simulink model "sampleModel1496_4"  (R2023a)
settings: Solver=VariableStepAuto  StartTime=0.0  StopTime=10.0  RelTol=1e-3
libraries: hdlsllib x6
settings Model: Creator=user1  LastModifiedBy=user1

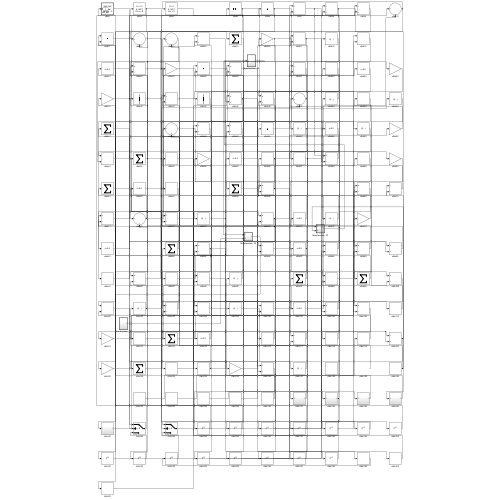
[thumbnail: Simulink's stored preview of the top-level diagram]
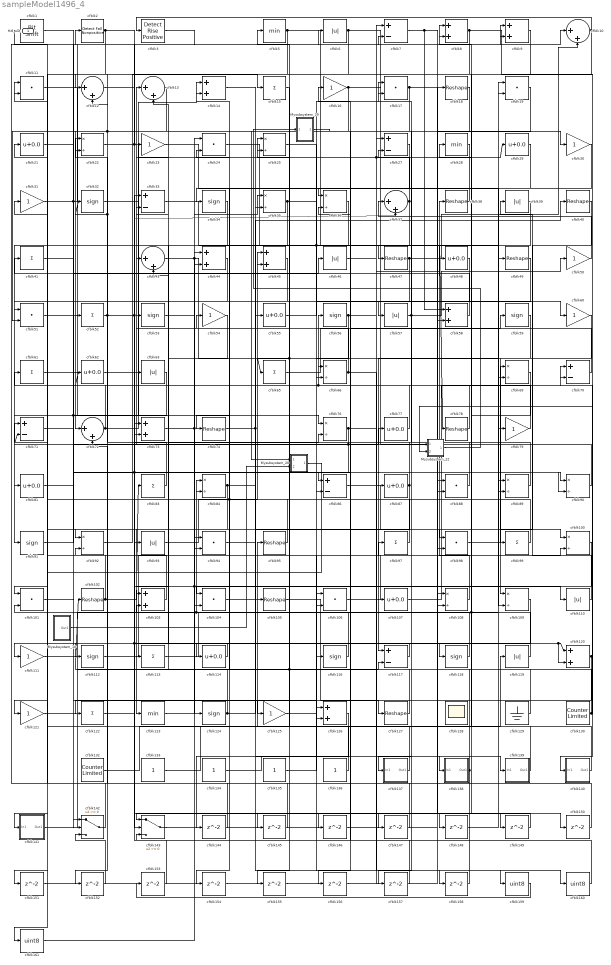
== system sampleModel1496_4 ==
  Mysubsystem_10 : Subsystem  TreatAsAtomicUnit=on  RTWFcnName=Mysubsystem_10
      settings: RTWFcnNameOpts=User specified  RTWFileNameOpts=Use function name
  Mysubsystem_20 : Subsystem  TreatAsAtomicUnit=on  RTWFcnName=Mysubsystem_20
      settings: RTWFcnNameOpts=User specified  RTWFileNameOpts=Use function name
  Mysubsystem_22 : Subsystem  TreatAsAtomicUnit=on  RTWFcnName=Mysubsystem_22
      settings: RTWFcnNameOpts=User specified  RTWFileNameOpts=Use function name
  Mysubsystem_29 : Subsystem  TreatAsAtomicUnit=on  RTWFcnName=Mysubsystem_29
      settings: RTWFcnNameOpts=User specified  RTWFileNameOpts=Use function name
  cfblk1 : hdlsllib/Logic and Bit Operations/Bit Shift  mode=Shift Left Logical  N=0
  cfblk{10,12..13,37,43,72} (6 alike) : Sum  Inputs=|++  OutDataTypeStr=uint8
  cfblk{22,25,35..36,66,69,76,84,89..90,92,100,108..109} (14 alike) : Product  Inputs=*/  OutDataTypeStr=uint8  RndMeth=Zero  SaturateOnIntegerOverflow=on
  cfblk{11,17,19,24,51,88,94,98,101,104,106} (11 alike) : DotProduct  OutDataTypeStr=uint8
  cfblk{18,38,40,47,49,74,78,95,102,105,127} (11 alike) : Reshape
  cfblk{8..9,14,44..45,58,73,103,120,126} (10 alike) : Sum  OutDataTypeStr=uint8
  cfblk{21,29,48,55,62,77,81,87,107,114} (10 alike) : Bias  Bias=0.0  SaturateOnIntegerOverflow=off
  cfblk{6,39,46,57,63,93,110,119} (8 alike) : Abs  OutDataTypeStr=uint8  SaturateOnIntegerOverflow=off
  cfblk{16,23,30..31,50,54,60,79,111,121,125} (11 alike) : Gain  OutDataTypeStr=uint8
  cfblk{32,34,53,56,59,91,112,116,118,124} (10 alike) : Signum
  cfblk{15,41,52,61,65,83,97,99,113,122} (10 alike) : Sum  Inputs=+  OutDataTypeStr=uint8
  cfblk{7,27,33,70..71,86,117} (7 alike) : Sum  Inputs=+-  OutDataTypeStr=uint8
  cfblk123 : MinMax  OutDataTypeStr=uint8
  cfblk128 : Scope
      settings: Floating=on
  cfblk129 : Ground
  cfblk130 : hdlsllib/Sources/Counter Limited  uplimit=7  tsamp=-1
  cfblk132 : hdlsllib/Sources/Counter Limited  uplimit=7  tsamp=-1
  cfblk{133..136} (4 alike) : Constant  OutDataTypeStr=uint8  SampleTime=-1
  cfblk137 : Subsystem
      settings: LibrarySourceBlock=|
      | hdlsllib/Ports &
      | Subsystems/Subsystem
  cfblk138 : Subsystem
      settings: LibrarySourceBlock=|
      | hdlsllib/Ports &
      | Subsystems/Subsystem
  cfblk139 : Subsystem
      settings: LibrarySourceBlock=|
      | hdlsllib/Ports &
      | Subsystems/Subsystem
  cfblk140 : Subsystem
      settings: LibrarySourceBlock=|
      | hdlsllib/Ports &
      | Subsystems/Subsystem
  cfblk141 : Subsystem
      settings: LibrarySourceBlock=|
      | hdlsllib/Ports &
      | Subsystems/Subsystem
  cfblk142 : Switch  OutDataTypeStr=uint8  SaturateOnIntegerOverflow=off  InputSameDT=off
  cfblk143 : Switch  OutDataTypeStr=uint8  SaturateOnIntegerOverflow=off  InputSameDT=off
  cfblk{144..158} (15 alike) : Delay  SampleTime=1
  cfblk159 : DataTypeConversion  OutDataTypeStr=uint8  SaturateOnIntegerOverflow=off  RndMeth=Floor
  cfblk160 : DataTypeConversion  OutDataTypeStr=uint8  SaturateOnIntegerOverflow=off  RndMeth=Floor
  cfblk161 : DataTypeConversion  OutDataTypeStr=uint8  SaturateOnIntegerOverflow=off  RndMeth=Floor
  cfblk2 : hdlsllib/Logic and Bit Operations/Detect Fall Nonpositive  vinit=0  OutDataTypeStr=uint8
  cfblk28 : MinMax  OutDataTypeStr=uint8
  cfblk3 : hdlsllib/Logic and Bit Operations/Detect Rise Positive  vinit=0  OutDataTypeStr=uint8
  cfblk5 : MinMax  OutDataTypeStr=uint8
  Hdl_out : Outport  OutDataTypeStr=uint8
  wires:
  cfblk90/1 -> cfblk13/1
  cfblk92/1 -> cfblk15/1
  cfblk123/1 -> cfblk44/1
  cfblk108/1 -> cfblk38/1
  cfblk8/1 -> cfblk140/1(In1), cfblk121/1
  cfblk72/1 -> cfblk45/1, cfblk61/1
  cfblk59/1 -> cfblk109/1
  cfblk118/1 -> cfblk84/1, cfblk11/2
  cfblk39/1 -> cfblk91/1
  cfblk65/1 -> cfblk59/1
  cfblk87/1 -> cfblk123/1, cfblk25/2
  cfblk142/1 -> cfblk2/1
  cfblk102/1 -> cfblk83/1, cfblk11/1
  cfblk22/1 -> cfblk124/1, cfblk9/1
  cfblk17/1 -> cfblk72/1, cfblk30/1
  cfblk5/1 -> cfblk47/1, cfblk122/1
  cfblk51/1 -> cfblk93/1
  cfblk6/1 -> cfblk109/2, cfblk12/1
  cfblk60/1 -> cfblk117/1
  cfblk45/1 -> cfblk74/1
  cfblk3/1 -> cfblk7/2
  cfblk107/1 -> cfblk70/1
  cfblk1/1 -> cfblk73/2, cfblk90/1
  cfblk27/1 -> cfblk36/1
  cfblk93/1 -> cfblk45/2
  cfblk62/1 -> cfblk14/1
  cfblk61/1 -> cfblk76/1
  cfblk31/1 -> cfblk6/1, cfblk8/2
  cfblk89/1 -> cfblk53/1
  cfblk49/1 -> cfblk57/1
  cfblk11/1 -> cfblk126/1
  cfblk70/1 -> cfblk16/1
  cfblk84/1 -> cfblk101/1, cfblk108/2
  cfblk98/1 -> cfblk69/1
  cfblk46/1 -> cfblk29/1, cfblk9/2
  cfblk117/1 -> cfblk111/1
  cfblk127/1 -> cfblk102/1, cfblk25/1
  cfblk43/1 -> cfblk89/1, cfblk87/1
  cfblk140/1(Out1) -> cfblk95/1
  cfblk15/1 -> cfblk65/1, cfblk155/1
  cfblk24/1 -> cfblk78/1, cfblk66/2
  cfblk58/1 -> cfblk41/1
  cfblk16/1 -> Mysubsystem_22/1(In1), cfblk35/2
  cfblk19/1 -> cfblk86/1
  cfblk104/1 -> cfblk55/1
  cfblk52/1 -> cfblk110/1, cfblk90/2, cfblk37/2, cfblk22/1
  cfblk79/1 -> cfblk23/1
  cfblk57/1 -> cfblk50/1, cfblk137/1(In1)
  cfblk116/1 -> cfblk14/2
  cfblk141/1(Out1) -> cfblk44/2
  cfblk78/1 -> cfblk56/1, cfblk62/1
  cfblk63/1 -> cfblk81/1
  cfblk134/1 -> cfblk138/1(In1)
  cfblk77/1 -> cfblk54/1
  cfblk7/1 -> cfblk58/1, cfblk149/1
  cfblk105/1 -> cfblk127/1
  cfblk143/1 -> cfblk88/1
  cfblk13/1 -> cfblk92/1, cfblk51/2
  cfblk10/1 -> cfblk3/1, cfblk12/2
  cfblk33/1 -> cfblk116/1
  cfblk125/1 -> cfblk97/1
  cfblk14/1 -> cfblk98/1
  cfblk120/1 -> Mysubsystem_22/2(In2), cfblk152/1
  cfblk66/1 -> cfblk43/1, cfblk158/1
  cfblk21/1 -> cfblk52/1
  cfblk129/1 -> cfblk84/2
  cfblk122/1 -> cfblk76/2
  cfblk95/1 -> cfblk71/1
  cfblk91/1 -> cfblk77/1
  cfblk81/1 -> cfblk46/1
  cfblk130/1 -> cfblk70/2, cfblk43/2
  cfblk56/1 -> cfblk86/2, cfblk60/1
  cfblk139/1(Out1) -> cfblk28/1
  cfblk99/1 -> cfblk31/1
  cfblk112/1 -> cfblk18/1
  cfblk54/1 -> cfblk103/1
  cfblk35/1 -> cfblk104/1, cfblk58/2
  cfblk111/1 -> cfblk19/1
  cfblk38/1 -> cfblk34/1
  cfblk71/1 -> cfblk10/1
  cfblk73/1 -> cfblk125/1, cfblk106/2, cfblk35/1
  cfblk69/1 -> cfblk118/1
  cfblk103/1 -> cfblk92/2
  cfblk34/1 -> cfblk113/1
  cfblk86/1 -> cfblk100/1
  cfblk76/1 -> cfblk71/2, cfblk142/2, cfblk48/1
  cfblk44/1 -> cfblk104/2
  cfblk113/1 -> cfblk79/1
  cfblk37/1 -> cfblk27/2, cfblk141/1(In1)
  cfblk110/1 -> cfblk39/1
  cfblk136/1 -> cfblk5/1
  cfblk119/1 -> cfblk13/2, cfblk8/1
  cfblk36/1 -> cfblk143/2
  cfblk132/1 -> cfblk119/1
  cfblk135/1 -> cfblk106/1
  cfblk41/1 -> cfblk142/1
  cfblk47/1 -> cfblk10/2, cfblk51/1
  cfblk23/1 -> cfblk49/1
  cfblk50/1 -> cfblk37/1
  cfblk30/1 -> cfblk114/1
  cfblk40/1 -> cfblk99/1
  cfblk2/1 -> cfblk120/1, cfblk120/2, cfblk150/1, cfblk161/1
  cfblk124/1 -> cfblk117/2, cfblk103/2
  cfblk114/1 -> cfblk112/1
  cfblk32/1 -> cfblk19/2
  cfblk106/1 -> cfblk100/2
  cfblk133/1 -> cfblk89/2
  cfblk55/1 -> cfblk17/1
  cfblk138/1(Out1) -> cfblk143/3, cfblk66/1
  cfblk88/1 -> cfblk17/2
  cfblk137/1(Out1) -> cfblk21/1
  cfblk121/1 -> cfblk105/1
  cfblk83/1 -> cfblk32/1, cfblk22/2
  cfblk74/1 -> cfblk139/1(In1), cfblk40/1
  cfblk97/1 -> cfblk33/2, cfblk24/2
  cfblk101/1 -> cfblk126/2
  cfblk12/1 -> cfblk63/1
  cfblk53/1 -> cfblk107/1
  cfblk126/1 -> cfblk144/1
  cfblk144/1 -> cfblk101/2
  cfblk28/1 -> cfblk145/1
  cfblk145/1 -> cfblk1/1
  cfblk109/1 -> cfblk146/1
  cfblk146/1 -> cfblk108/1
  cfblk29/1 -> cfblk147/1
  cfblk147/1 -> cfblk73/1
  cfblk9/1 -> cfblk148/1
  cfblk148/1 -> cfblk69/2
  cfblk149/1 -> cfblk143/1
  cfblk150/1 -> cfblk72/2
  cfblk151/1 -> cfblk7/1
  cfblk152/1 -> cfblk142/3
  cfblk153/1 -> cfblk33/1
  cfblk100/1 -> cfblk154/1
  cfblk154/1 -> cfblk98/2
  cfblk155/1 -> cfblk88/2
  cfblk48/1 -> cfblk156/1
  cfblk156/1 -> cfblk27/1
  cfblk18/1 -> cfblk157/1
  cfblk157/1 -> cfblk36/2
  cfblk158/1 -> cfblk24/1
  cfblk94/1 -> cfblk159/1
  cfblk159/1 -> cfblk153/1
  cfblk25/1 -> cfblk160/1
  cfblk160/1 -> cfblk94/1
  cfblk161/1 -> cfblk94/2
  Mysubsystem_10/1(Out1) -> Mysubsystem_20/2(In2)
  Mysubsystem_20/1(Out1) -> cfblk151/1
  Mysubsystem_22/1(Out1) -> Mysubsystem_29/1(In1)
  Mysubsystem_29/1(Out1) -> Mysubsystem_20/1(In1)

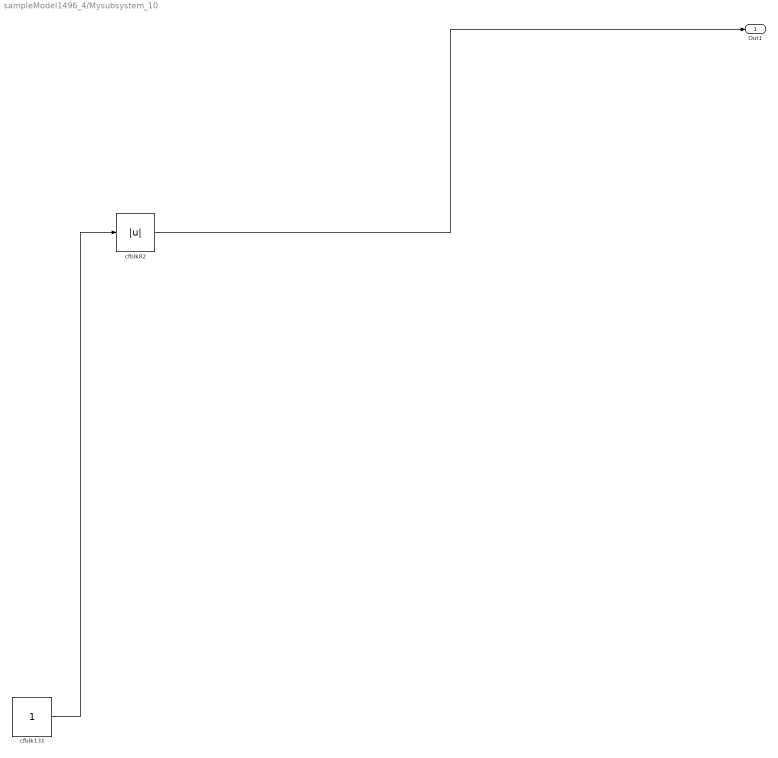
== system sampleModel1496_4/Mysubsystem_10 ==
  cfblk131 : Constant  SampleTime=-1
  cfblk82 : Abs  SaturateOnIntegerOverflow=off
  Out1 : Outport
  wires:
  cfblk131/1 -> cfblk82/1
  cfblk82/1 -> Out1/1

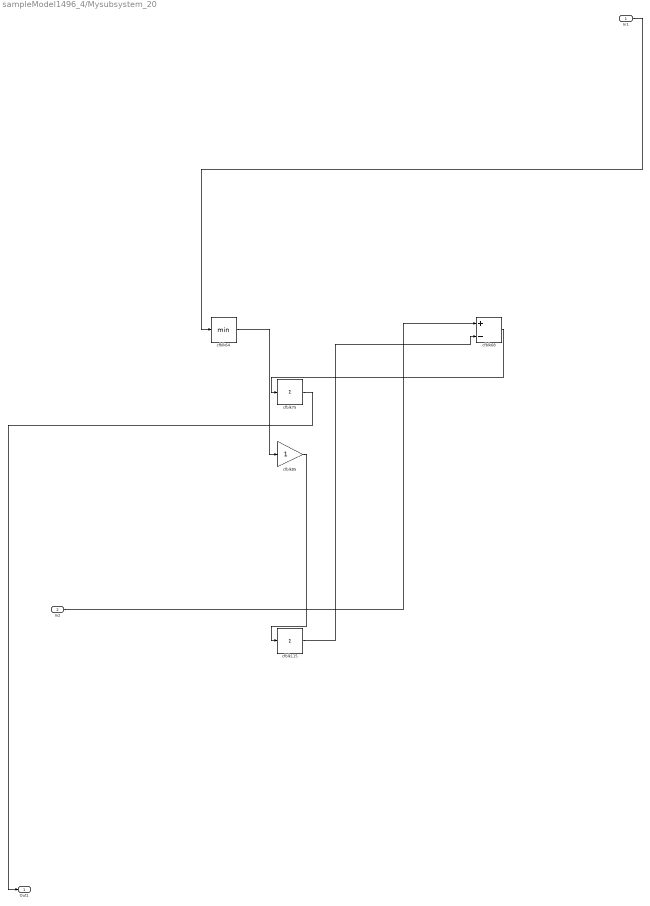
== system sampleModel1496_4/Mysubsystem_20 ==
  In1 : Inport
  In2 : Inport  Port=2
  cfblk115 : Sum  Inputs=+
  cfblk64 : MinMax
  cfblk68 : Sum  Inputs=+-
  cfblk75 : Sum  Inputs=+
  cfblk85 : Gain
  Out1 : Outport
  wires:
  cfblk115/1 -> cfblk68/2
  cfblk64/1 -> cfblk85/1
  In1/1 -> cfblk64/1
  cfblk75/1 -> Out1/1
  cfblk85/1 -> cfblk115/1
  cfblk68/1 -> cfblk75/1
  In2/1 -> cfblk68/1

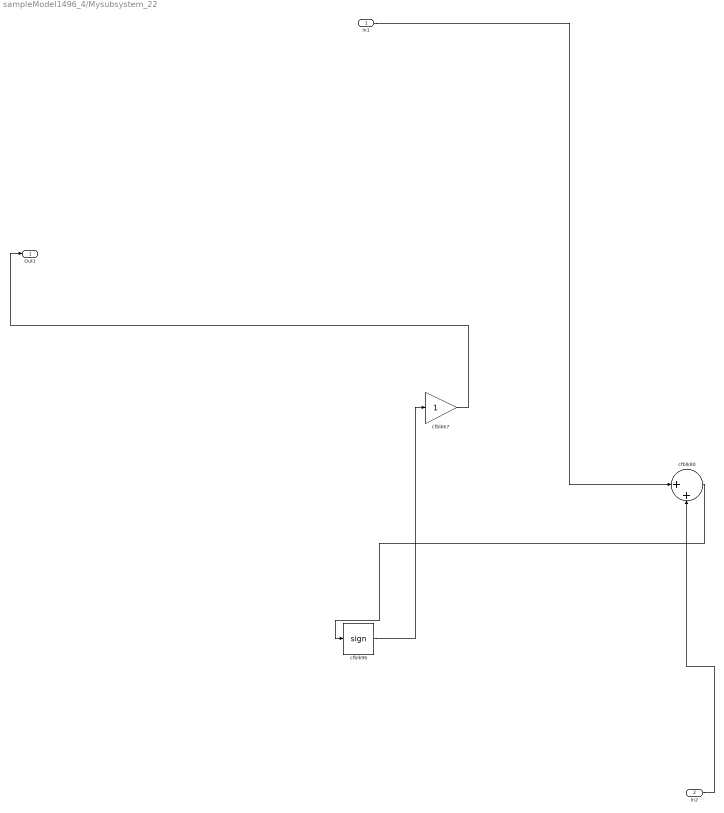
== system sampleModel1496_4/Mysubsystem_22 ==
  In1 : Inport
  In2 : Inport  Port=2
  cfblk67 : Gain
  cfblk80 : Sum  Inputs=|++
  cfblk96 : Signum
  Out1 : Outport
  wires:
  cfblk80/1 -> cfblk96/1
  cfblk96/1 -> cfblk67/1
  In2/1 -> cfblk80/2
  cfblk67/1 -> Out1/1
  In1/1 -> cfblk80/1

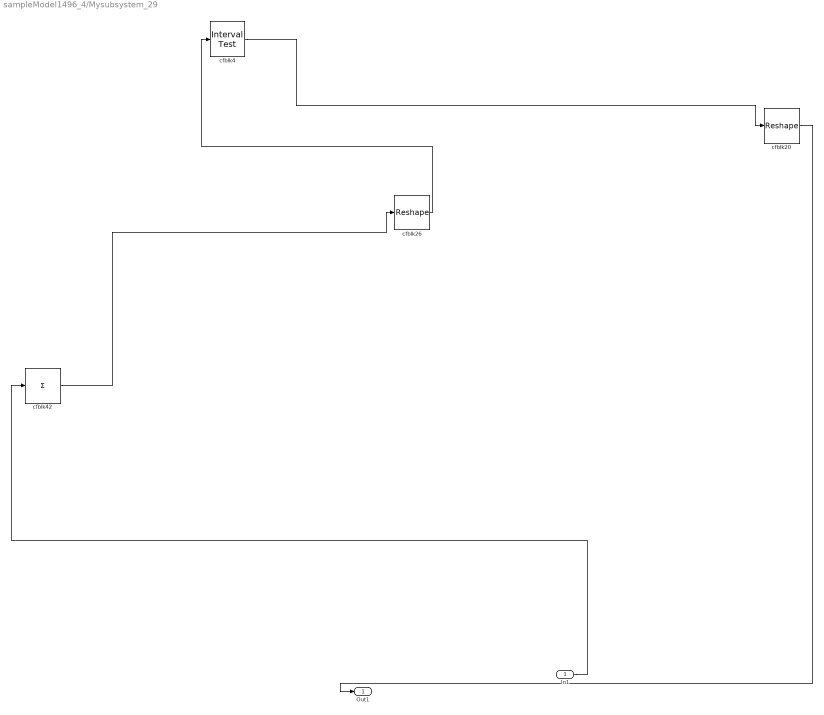
== system sampleModel1496_4/Mysubsystem_29 ==
  In1 : Inport
  cfblk20 : Reshape
  cfblk26 : Reshape
  cfblk4 : hdlsllib/Logic and Bit Operations/Interval Test  IntervalClosedRight=on  uplimit=0.5  IntervalClosedLeft=on  lowlimit=-0.5  OutDataTypeStr=boolean
  cfblk42 : Sum  Inputs=+
  Out1 : Outport
  wires:
  cfblk4/1 -> cfblk20/1
  cfblk26/1 -> cfblk4/1
  cfblk42/1 -> cfblk26/1
  cfblk20/1 -> Out1/1
  In1/1 -> cfblk42/1

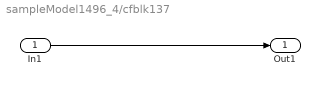
== system sampleModel1496_4/cfblk137 ==
  In1 : Inport
  Out1 : Outport
  wires:
  In1/1 -> Out1/1

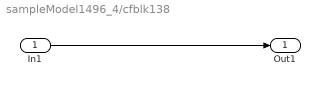
== system sampleModel1496_4/cfblk138 ==
  In1 : Inport
  Out1 : Outport
  wires:
  In1/1 -> Out1/1

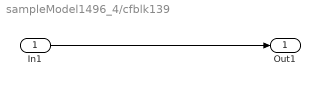
== system sampleModel1496_4/cfblk139 ==
  In1 : Inport
  Out1 : Outport
  wires:
  In1/1 -> Out1/1

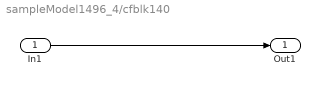
== system sampleModel1496_4/cfblk140 ==
  In1 : Inport
  Out1 : Outport
  wires:
  In1/1 -> Out1/1

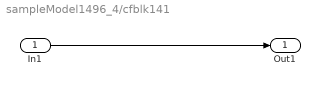
== system sampleModel1496_4/cfblk141 ==
  In1 : Inport
  Out1 : Outport
  wires:
  In1/1 -> Out1/1
